simulink model "Elektrownia_simulink"  (R2016a)
settings: Solver=VariableStepAuto  StartTime=0.0  StopTime=100  RelTol=1e-3
values from neighbouring files (symbols this model uses):
  A_pr = 4.52    [Elektrownia.m]
  C_lp_sg = 3809.9    [Elektrownia.m]
  C_p_pc = 5355    [Elektrownia.m]
  C_p_pr = 6873.1    [Elektrownia.m]
  C_psi = 13.75 * (10 ^ 6)    (= 13750000)    [Elektrownia.m]
  C_vp_sg = 3635.6    [Elektrownia.m]
  E_evap_sg = 1.658 * (10 ^ 6)    (= 1658000)    [Elektrownia.m]
  Kt_sg = 9.5296*(10^6)    (= 9529600)    [Elektrownia.m]
  LAMBDA = 10 ^ -5    (= 1e-05)    [Elektrownia.m]
  M_in = 1.4222    [Elektrownia.m]
  M_out = 2.11    [Elektrownia.m]
  m_sg = 119.31    [Elektrownia.m]
  M_sg = 34920    [Elektrownia.m]
  P_1 = -1.223e-4    (= -0.0001223)    [Elektrownia.m]
  P_2 = -5.502e-5    (= -5.502e-05)    [Elektrownia.m]
  P_3 = -1.953e-4    (= -0.0001953)    [Elektrownia.m]
  S = 1938.9    [Elektrownia.m]
  T_pc_hl = 296.13    [Elektrownia.m]
  T_pc_i = 258.85    [Elektrownia.m]
  T_sg_sw = 220.85    [Elektrownia.m]
  V = 0    [Elektrownia.m]
  V_0_pc = 242    [Elektrownia.m]
  W_loss_pc = 2.996 * (10 ^ 7)    (= 29960000)    [Elektrownia.m]
  W_loss_pr = 1.6823 * (10 ^ 5)    (= 168230)    [Elektrownia.m]
  W_loss_sg = 1.8932  * (10 ^ 7)    (= 18932000)    [Elektrownia.m]
undefined symbols (not defined in the file or in its folder): W_heat_pr, X_mpr_gtz, X_mpr_ltz
settings Model: Creator=Michal Chruscinski  LastModifiedBy=Michal Chruscinski

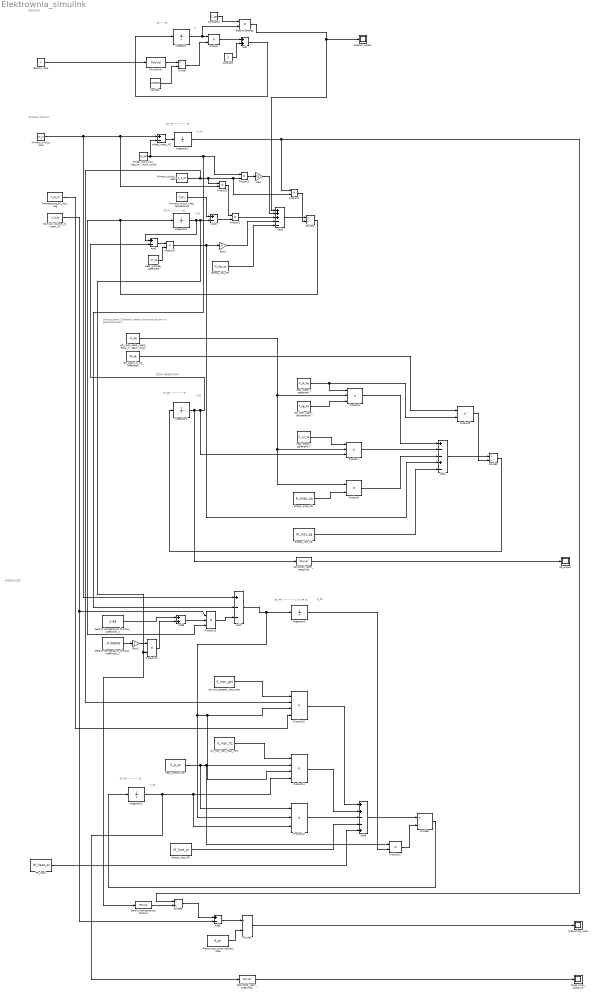
== system Elektrownia_simulink ==
  note: dM_PC
      | ------------
      |      dt
  note: M_PC
  note: T_SG
  note: dT_SG
      | ------------
      |     dt
  note: N
  note: dN
      | ----
      | dt
  note: PRESSURIZER
  note: dT_PR
      | -----------
      |     dt
  note: T_PR
  note: dT_PC
      | -----------
      |     dt
  note: T_PC
  note: dM_PR
      | ------------ = m_PR
      |     dt
  note: M_PR
  note: PRIMARY CIRCUIT
  note: REACTOR
  note: STEAM GENERATOR
  note: Uproszczenie! Zakladamy idealny sterownik
      | poziomu w generatorze pary!
  Add : Sum
  Add1 : Sum  Inputs=+-
  Add2 : Sum  Inputs=+-
  Add3 : Sum  Inputs=+++--
  Add4 : Sum  Inputs=+--+-
  Add5 : Sum  Inputs=++--+
  Add6 : Sum  Inputs=+-
  Add7 : Sum  Inputs=+--
  Add8 : Sum
  Constant : Constant  Value=S
  Constant1 : Constant  Value=C_psi
  Density-temperature_function : Polyval  Coefs=[-0.00848, 2.98, 581.2]
  Density-temperature_function_coefficient_1 : Constant  Value=2.98
  Density-temperature_function_coefficient_2 : Constant  Value=-0.00848
  Divide{,1..5} (6 alike) : Product  Inputs=*/
  Energy_evap_SG : Constant  Value=E_evap_sg
  Energy_loss_PR : Constant  Value=W_loss_pr
  Energy_lost_PC : Constant  Value=W_loss_pc
  Energy_lost_SG : Constant  Value=W_loss_sg
  Gain : Gain  Gain=15
  Gain1 : Gain  Gain=6
  Gain2 : Gain  Gain=2
  Heat_transfer_coefficient : Constant  Value=Kt_sg
  Integrator{,1..5} (6 alike) : Integrator
  Lambda : Constant  Value=LAMBDA
  Nominal_volume_of_water_PC : Constant  Value=V_0_pc
  PR_input : Constant  Value=W_heat_pr
  Polynomial : Polyval  Coefs=[P_1, P_2, P_3]
  Pressurizer_cross-section_area : Constant  Value=A_pr
  Pressurizer_level : Scope
  Pressurizer_pressure : Scope
  Primary_circuit_heat : Constant  Value=C_p_pc
  Primary_circuit_inlet_temperature : Constant  Value=T_pc_i
  Primary_circuit_input : Constant  Value=M_in
  Product{,1..5,8..9,14..15} (10 alike) : Product
  Product10 : Product  Inputs=4
  Product11 : Product  Inputs=4
  Product{6..7,12..13} (4 alike) : Product  Inputs=3
  "Purge_mass_flow_rate_primary_circuit " : Constant  Value=M_out
  Reactor_energy : Product
  Reactor_output : Scope
  SG_inlet_water_mass_equal_to_outlet_steam_mass : Constant  Value=m_sg
  SG_inlet_water_temperature : Constant  Value=T_sg_sw
  SG_mass_in_out_difference : Constant  Value=M_sg
  SG_output : Scope
  Saturated_vapor_pressure1 : Polyval  Coefs=[0.63, -258.01, 28884.78]
  Saturated_vapor_pressure2 : Polyval  Coefs=[0.63, -258.01, 28884.78]
  Temperature_PC_Hot_Leg : Constant  Value=T_pc_hl
  Water_mass_PC : Sum  Inputs=+-
  chi_mpr_greater_than_zero : Constant  Value=X_mpr_gtz
  chi_mpr_less_than_zero : Constant  Value=X_mpr_ltz
  hear_pressurizer : Constant  Value=C_p_pr
  heat_steam_generator : Constant  Value=C_lp_sg
  heat_steam_generator1 : Constant  Value=C_vp_sg
  "reactor_input " : Constant  Value=V
  wires:
  Integrator/1 -> Reactor_energy/2, Product/1
  Product/1 -> Add/1
  Constant/1 -> Add/2
  Add/1 -> Integrator/1
  "reactor_input "/1 -> Polynomial/1
  Polynomial/1 -> Divide/1
  Lambda/1 -> Divide/2
  Divide/1 -> Product/2
  Constant1/1 -> Reactor_energy/1
  Reactor_energy/1 -> Add3/1, Reactor_output/1
  Primary_circuit_input/1 -> Add7/1, Water_mass_PC/1, Product2/2
  "Purge_mass_flow_rate_primary_circuit "/1 -> Water_mass_PC/2, Add7/2, Product3/1
  Water_mass_PC/1 -> Integrator2/1
  Integrator1/1 -> Add1/1, Density-temperature_function/1, Product14/2, Add2/2
  Primary_circuit_inlet_temperature/1 -> Add2/1
  Add2/1 -> Product1/2
  Product2/1 -> Product1/1
  Primary_circuit_heat/1 -> Product10/2, Product2/1, Product4/2, Product3/2
  Product1/1 -> Add3/3
  Product3/1 -> Gain/1
  Gain/1 -> Add3/2
  Product5/1 -> Add4/4, Gain1/1
  Gain1/1 -> Add3/4
  Add3/1 -> Divide1/1
  Integrator2/1 -> Divide5/1, Product4/1
  Product4/1 -> Divide1/2
  Divide1/1 -> Integrator1/1, Product13/3
  Heat_transfer_coefficient/1 -> Product5/2
  Add1/1 -> Product5/1
  Energy_lost_PC/1 -> Add3/5
  heat_steam_generator/1 -> Product9/2, Product6/1
  SG_inlet_water_mass_equal_to_outlet_steam_mass/1 -> Product8/1, Product7/2, Product6/2
  SG_inlet_water_temperature/1 -> Product6/3
  heat_steam_generator1/1 -> Product7/1
  Integrator4/1 -> Saturated_vapor_pressure1/1, Add1/2, Product7/3
  Energy_evap_SG/1 -> Product8/2
  Product6/1 -> Add4/1
  Product7/1 -> Add4/2
  Product8/1 -> Add4/3
  Energy_lost_SG/1 -> Add4/5
  Add4/1 -> Divide2/1
  SG_mass_in_out_difference/1 -> Product9/1
  Product9/1 -> Divide2/2
  Divide2/1 -> Integrator4/1
  Temperature_PC_Hot_Leg/1 -> Product10/4
  chi_mpr_greater_than_zero/1 -> Product10/1
  Add7/1 -> Product10/3, Product11/3, Product12/2, Integrator5/1
  chi_mpr_less_than_zero/1 -> Product11/1
  hear_pressurizer/1 -> Product12/1, Product11/2, Product15/1
  Integrator3/1 -> Saturated_vapor_pressure2/1, Product12/3, Product11/4
  Product10/1 -> Add5/1
  Product11/1 -> Add5/2
  Product12/1 -> Add5/3
  Energy_loss_PR/1 -> Add5/4
  PR_input/1 -> Add5/5
  Product13/1 -> Add7/3
  Nominal_volume_of_water_PC/1 -> Add6/2, Product13/1
  Add8/1 -> Product13/2
  Density-temperature_function_coefficient_1/1 -> Add8/1
  Product14/1 -> Add8/2
  Density-temperature_function_coefficient_2/1 -> Gain2/1
  Gain2/1 -> Product14/1
  Add5/1 -> Divide3/1
  Product15/1 -> Divide3/2
  Integrator5/1 -> Product15/2
  Divide3/1 -> Integrator3/1
  Saturated_vapor_pressure1/1 -> SG_output/1
  Add6/1 -> Divide4/1
  Pressurizer_cross-section_area/1 -> Divide4/2
  Density-temperature_function/1 -> Divide5/2
  Divide5/1 -> Add6/1
  Divide4/1 -> Pressurizer_level/1
  Saturated_vapor_pressure2/1 -> Pressurizer_pressure/1
